simulink model "secondOrderUnityNegativeFeedbackSystem"  (R2021b)
settings: Solver=VariableStepAuto  StartTime=0.0  StopTime=10.0  RelTol=1e-3
libraries: cstblocks x5
settings Model: Creator=PRANAV ARYA  LastModifiedBy=PRANAV ARYA

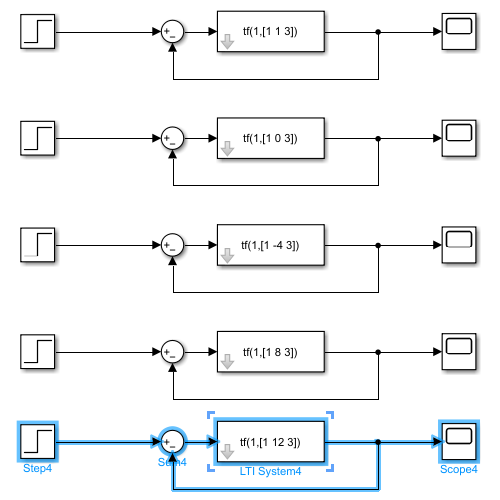
[thumbnail: Simulink's stored preview of the top-level diagram]
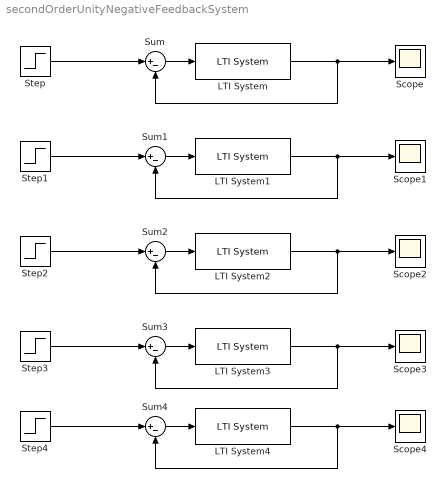
== system secondOrderUnityNegativeFeedbackSystem ==
  LTI System : cstblocks/LTI System  sys=tf(1,[1 1 3])  IC=[]
  LTI System1 : cstblocks/LTI System  sys=tf(1,[1 0 3])  IC=[]
  LTI System2 : cstblocks/LTI System  sys=tf(1,[1 -4 3])  IC=[]
  LTI System3 : cstblocks/LTI System  sys=tf(1,[1 8 3])  IC=[]
  LTI System4 : cstblocks/LTI System  sys=tf(1,[1 12 3])  IC=[]
  Scope{,1..4} (5 alike) : Scope
  Step{,1..4} (5 alike) : Step  SampleTime=0
  Sum{,1..4} (5 alike) : Sum  Inputs=|+-
  wires:
  Sum/1 -> LTI System/1
  Step/1 -> Sum/1
  LTI System/1 -> Sum/2, Scope/1
  Step1/1 -> Sum1/1
  LTI System1/1 -> Sum1/2, Scope1/1
  Sum1/1 -> LTI System1/1
  Sum3/1 -> LTI System3/1
  LTI System3/1 -> Sum3/2, Scope3/1
  Step3/1 -> Sum3/1
  Step2/1 -> Sum2/1
  Sum2/1 -> LTI System2/1
  LTI System2/1 -> Sum2/2, Scope2/1
  Sum4/1 -> LTI System4/1
  LTI System4/1 -> Sum4/2, Scope4/1
  Step4/1 -> Sum4/1
